simulink subsystem "HVAC_ECU"  (R2021a)
settings: Solver=VariableStepAuto  StartTime=0.0  StopTime=10.0  RelTol=1e-3
settings Model: Creator=prasad  LastModifiedBy=Sai229

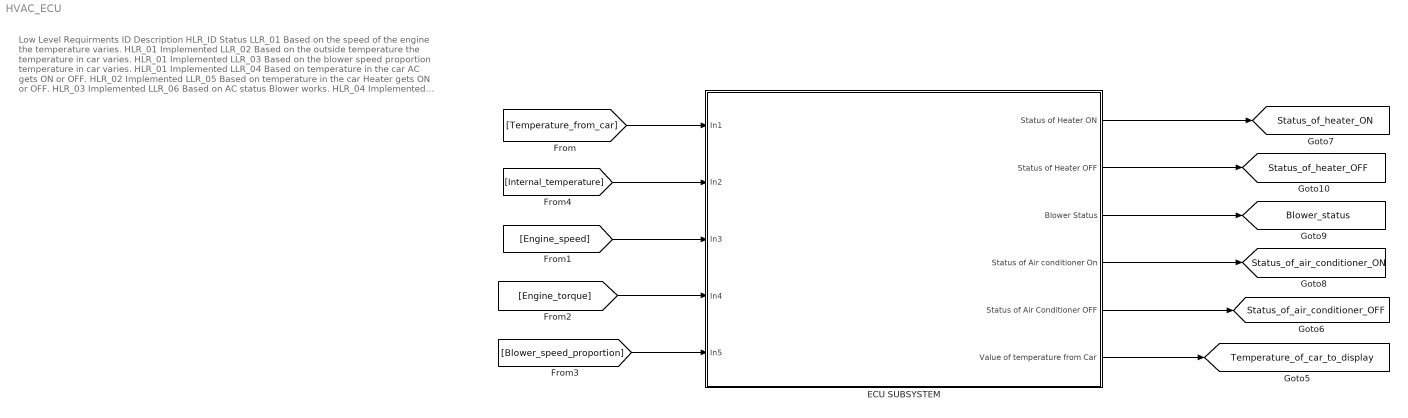
== system HVAC_ECU ==
  note: Low Level Requirments
      | ID
      | Description
      | HLR_ID
      | Status
      |
      | LLR_01
      | Based on the speed of the engine the temperature varies.
      | HLR_01
      | Implemented
      |
      | LLR_02
      | Based on the outside temperature the temperature in car varies.
      | HLR_01
      | Implemented
      |
      | LLR_03
      | Based on the blower speed proportion temperature in car varies.
      | HLR_01
      | Implemented
      |
      | LLR_04
      | Based on temperature in the car AC gets ON or OFF.
      | HLR_02
      | Implemented
      |
      | LLR_05
      | Based on temperature in the car Heater gets ON or OFF.
      | HLR_03
      | Implemented
      |
      | LLR_06
      | Based on AC status Blower works.
      | HLR_04
      | Implemented
      |
      | LOGIC:
      | STEP 1. Taking values of engine temperature and comp Torque and multipled and given to efficiency(gain).
      | STEP 2. Blower speed proportion and given toMaximum flow rate(gain).
      | STEP 3. Both values were given to divide block.
      | STEP 4. Internal Temperature is in degrees and after it converted into kelvin.
      | STEP 5. Subtract of both values, then the temperature will display on the Display block.
      | 1.Based on temperature the AC is getting on.
      | a.If the value(temperature) is greater than 25 then AC should be on.
      | b.Else the AC should be off.
      | 2. Based on AC status Blower Works.
      | 3. Based on temperature the Blower is getting on.
      | a.If the value(temperature) is less than 18 then Heater should be on.
      | b.Else the Heater should be off.
  " ECU SUBSYSTEM" : Subsystem
  tag scope: Blower_status=global, Status_of_air_conditioner_OFF=global, Status_of_air_conditioner_ON=global, Status_of_heater_OFF=global, Status_of_heater_ON=global, Temperature_of_car_to_display=global
  wires:
  [Temperature_from_car] -> " ECU SUBSYSTEM"/1(In1)
  " ECU SUBSYSTEM"/2(Status of Heater OFF) -> [Status_of_heater_OFF]
  " ECU SUBSYSTEM"/4(Status of Air conditioner On) -> [Status_of_air_conditioner_ON]
  [Internal_temperature] -> " ECU SUBSYSTEM"/2(In2)
  " ECU SUBSYSTEM"/3(Blower Status) -> [Blower_status]
  [Engine_torque] -> " ECU SUBSYSTEM"/4(In4)
  [Engine_speed] -> " ECU SUBSYSTEM"/3(In3)
  " ECU SUBSYSTEM"/5(Status of Air Conditioner OFF) -> [Status_of_air_conditioner_OFF]
  [Blower_speed_proportion] -> " ECU SUBSYSTEM"/5(In5)
  " ECU SUBSYSTEM"/6(Value of temperature from Car) -> [Temperature_of_car_to_display]
  " ECU SUBSYSTEM"/1(Status of Heater ON) -> [Status_of_heater_ON]

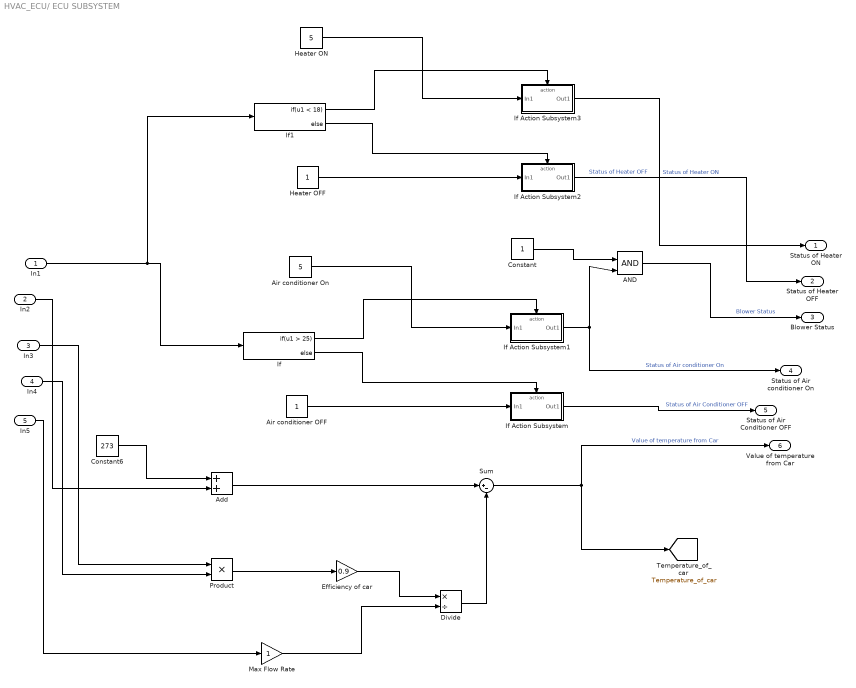
== system HVAC_ECU/ ECU SUBSYSTEM ==
  In1 : Inport
  In2 : Inport  Port=2
  In3 : Inport  Port=3
  In4 : Inport  Port=4
  In5 : Inport  Port=5
  AND : Logic  IconShape=distinctive  AllPortsSameDT=off  OutDataTypeStr=boolean
  Add : Sum
  Air conditioner OFF : Constant
  Air conditioner On : Constant  Value=5
  Constant : Constant
  Constant6 : Constant  Value=273
  Divide : Product  Inputs=*/
  Efficiency of car : Gain  Gain=0.9
  Heater OFF : Constant
  Heater ON : Constant  Value=5
  If : If  IfExpression=u1 > 25
  If Action Subsystem : Subsystem  TreatAsAtomicUnit=on
  If Action Subsystem1 : Subsystem  TreatAsAtomicUnit=on
  If Action Subsystem2 : Subsystem  TreatAsAtomicUnit=on
  If Action Subsystem3 : Subsystem  TreatAsAtomicUnit=on
  If1 : If  IfExpression=u1 < 18
  Max Flow Rate : Gain
  Product : Product
  Sum : Sum  Inputs=|+-
  Status of Heater ON : Outport
  Status of Heater OFF : Outport  Port=2
  Blower Status : Outport  Port=3
  Status of Air conditioner On : Outport  Port=4
  Status of Air Conditioner OFF : Outport  Port=5
  Value of temperature from Car : Outport  Port=6
  tag scope: Temperature_of_car=global
  wires:
  If Action Subsystem/1(Out1) -> Status of Air Conditioner OFF/1  "Status of Air Conditioner OFF"
  In2/1 -> Add/2
  In4/1 -> Product/2
  If Action Subsystem2/1(Out1) -> Status of Heater OFF/1  "Status of Heater OFF"
  In3/1 -> Product/1
  If Action Subsystem3/1(Out1) -> Status of Heater ON/1  "Status of Heater ON"
  Air conditioner On/1 -> If Action Subsystem1/1(In1)
  AND/1 -> Blower Status/1  "Blower Status"
  If/2 -> If Action Subsystem/Action
  In5/1 -> Max Flow Rate/1
  Constant6/1 -> Add/1
  If/1 -> If Action Subsystem1/Action
  Add/1 -> Sum/1
  Heater OFF/1 -> If Action Subsystem2/1(In1)
  Product/1 -> Efficiency of car/1
  Air conditioner OFF/1 -> If Action Subsystem/1(In1)
  Heater ON/1 -> If Action Subsystem3/1(In1)
  If1/2 -> If Action Subsystem2/Action
  Efficiency of car/1 -> Divide/1
  Max Flow Rate/1 -> Divide/2
  If1/1 -> If Action Subsystem3/Action
  Sum/1 -> [Temperature_of_car], Value of temperature from Car/1  "Value of temperature from Car"
  If Action Subsystem1/1(Out1) -> AND/2, Status of Air conditioner On/1  "Status of Air conditioner On"
  Constant/1 -> AND/1
  In1/1 -> If/1, If1/1
  Divide/1 -> Sum/2

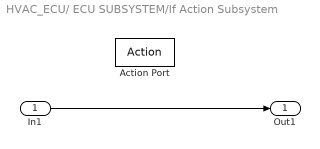
== system HVAC_ECU/ ECU SUBSYSTEM/If Action Subsystem ==
  In1 : Inport
  Action Port : ActionPort
  Out1 : Outport
  wires:
  In1/1 -> Out1/1

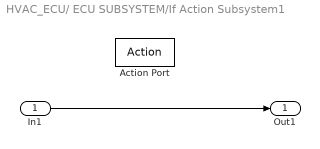
== system HVAC_ECU/ ECU SUBSYSTEM/If Action Subsystem1 ==
  In1 : Inport
  Action Port : ActionPort
  Out1 : Outport
  wires:
  In1/1 -> Out1/1

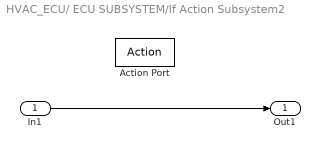
== system HVAC_ECU/ ECU SUBSYSTEM/If Action Subsystem2 ==
  In1 : Inport
  Action Port : ActionPort
  Out1 : Outport
  wires:
  In1/1 -> Out1/1

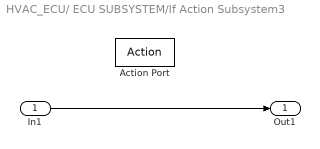
== system HVAC_ECU/ ECU SUBSYSTEM/If Action Subsystem3 ==
  In1 : Inport
  Action Port : ActionPort
  Out1 : Outport
  wires:
  In1/1 -> Out1/1
